simulink model "pendulum_simulation_simulank"  (R2022b)
settings: Solver=VariableStepAuto  StartTime=0.0  StopTime=10.0  MaxStep=.0001  RelTol=1e-3
values from neighbouring files (symbols this model uses):
  g = 9.81    [pendulum_simulation.m]
  L = LValue(i)    [pendulum_simulation.m]
settings Model: Creator=ahmed  LastModifiedBy=ahmed
settings DataIOCC: SaveFormat=StructureWithTime

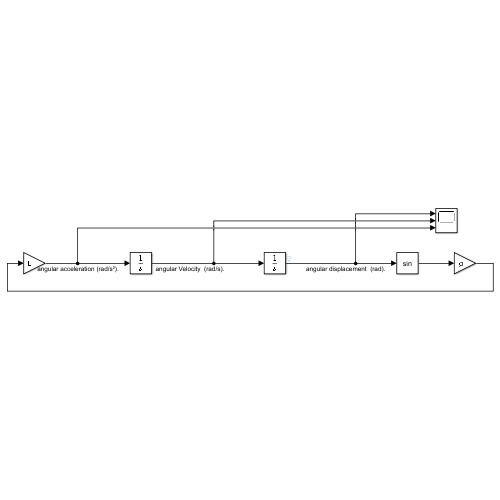
[thumbnail: Simulink's stored preview of the top-level diagram]
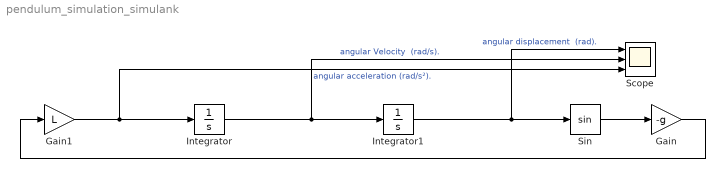
== system pendulum_simulation_simulank ==
  Gain : Gain  Gain=-g
  Gain1 : Gain  Gain=L
  Integrator : Integrator  InitialCondition=1
  Integrator1 : Integrator  InitialCondition=1
  Scope : Scope  NumInputPorts=3
  Sin : Trigonometry
  wires:
  Integrator1/1 -> Scope/1, Sin/1  "angular displacement  (rad)."
  Gain1/1 -> Scope/3, Integrator/1  "angular acceleration (rad/s²)."
  Integrator/1 -> Scope/2, Integrator1/1  "angular Velocity  (rad/s)."
  Sin/1 -> Gain/1
  Gain/1 -> Gain1/1
